simulink model "speed_model_validation_2"  (R2023b)
settings: Solver=FixedStepAuto  StartTime=0.0  StopTime=32  FixedStep=0.0001  MinStep=0.005  RelTol=1e-3  EnableMultiTasking=on
settings Model: SimulationMode=external  ExtModeTrigDuration=10  Creator=kiraa  LastModifiedBy=kiraa
settings OptimizationCC: EnhancedBackFolding=on  PassReuseOutputArgsThreshold=0  MaxStackSize=64  OptimizeBlockOrder=speed  DifferentSizesBufferReuse=on  OptimizationCustomize=off
settings DebuggingCC: ParameterTunabilityLossMsg=error
settings HardwareCC: ProdBitPerPointer=32  ProdBitPerSizeT=32  ProdBitPerPtrDiffT=32  ProdLargestAtomicInteger=Long  ProdLargestAtomicFloat=Double  ProdWordSize=32  ProdLongLongMode=on  ProdHWDeviceType=ARM Compatible->ARM Cortex
settings SFSimCC: MATLABDynamicMemAlloc=off
settings RTWCC: Toolchain=GNU Tools for ARM Embedded Processors
settings CodeAppCC: ForceParamTrailComments=on  OperatorAnnotations=on
settings GRTTargetCC: TargetLangStandard=C89/C90 (ANSI)

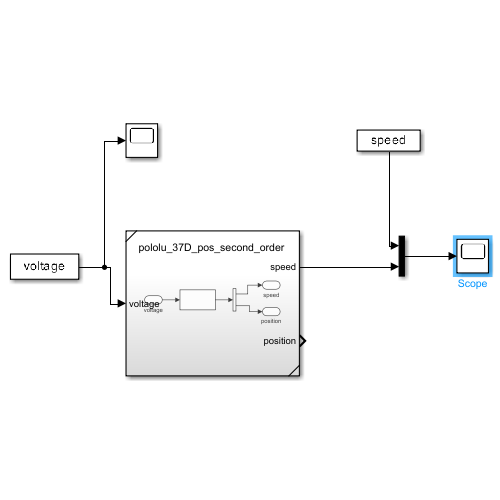
[thumbnail: Simulink's stored preview of the top-level diagram]
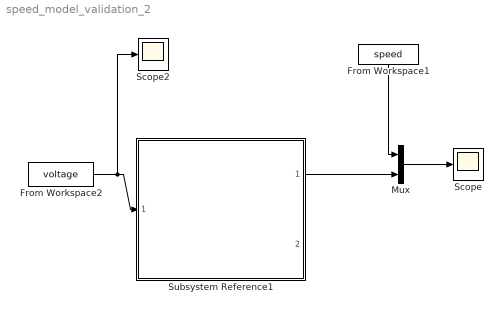
== system speed_model_validation_2 ==
  From Workspace1 : FromWorkspace  VariableName=speed
  From Workspace2 : FromWorkspace  VariableName=voltage
  Mux : Mux  Inputs=2
  Scope : Scope
  Scope2 : Scope
  Subsystem Reference1 : Subsystem  ReferencedSubsystem=pololu_37D_pos_second_order
  wires:
  From Workspace1/1 -> Mux/1
  Subsystem Reference1/1 -> Mux/2
  Mux/1 -> Scope/1
  From Workspace2/1 -> Scope2/1, Subsystem Reference1/1
